simulink model "ksp_zad16_1"  (Simulink 2.20)
settings: Solver=ode45  StartTime=0.0  StopTime=10.0  RelTol=1e-3  AbsTol=1e-6
undefined symbols (not defined in the file or in its folder): q0, q1, q2
settings Model: ConsistencyChecking=off  RTWPlaceOutputsASAP=off

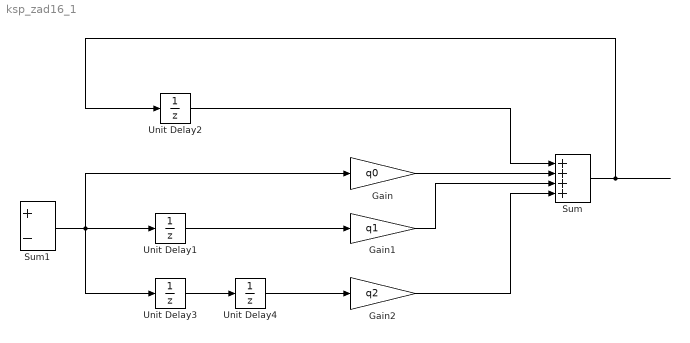
== system ksp_zad16_1 ==
  Gain : Gain  Gain=q0
  Gain1 : Gain  Gain=q1
  Gain2 : Gain  Gain=q2
  Sum : Sum  Inputs=++++
  Sum1 : Sum  Inputs=+-
  Unit Delay{1..4} (4 alike) : UnitDelay  X0=0  SampleTime=1
  wires:
  Gain2/1 -> Sum/4
  Unit Delay2/1 -> Sum/1
  Gain1/1 -> Sum/3
  Gain/1 -> Sum/2
  Sum1/1 -> Gain/1, Unit Delay1/1, Unit Delay3/1
  Unit Delay4/1 -> Gain2/1
  Unit Delay3/1 -> Unit Delay4/1
  Unit Delay1/1 -> Gain1/1
  Sum/1 -> Unit Delay2/1
